simulink model "QuerDynamicModell"  (R2018b)
settings: Solver=VariableStepAuto  StartTime=0.0  StopTime=10.0  RelTol=1e-3
model workspace (MAT data in the model file):
  chStern = 20.5517740291
  controllerActive = 0
  cvStern = 205.517740291
  deltaH = [0 0.02 0.04 0.06 0.08 0.1 0.12 0.14 0.16 0.18 0.2 0.22 0.24 0.26 0.28 0.3 0.32 0.34 0.36 0.38 0.4 0.42 0.44 0.46 0.48 0.5 0.52 0.54 0.56 0.58 0.6 0.62 0.64 0.66 0.68 0.7 0.72 0.74 0.76 0.78 0.8 0.82 0.84 0.86 0.88 0.9 0.92 0.94 0.96 0.98 1 1.02 1.04 1.06 1.08 1.1 1.12 1.14 1.16 1.18 1.2 1.22 1.24 1.26 1.28 1.3 1.32 1.34 1.36 1.38 1.4 1.42 1.44 1.46 1.48 1.5 1.52 1.54 1.56 1.58 1.6 1.62 1.64 1.66 1.68 1.7 1.72 1.74 1.76 1.78 1.8 1.82 1.84 1.86 1.88 1.9 1.92 1.94 1.96 1.98 2 2.02 2.04 2.06 2.08 2.1 2.12 2.14 2.16 2.18 2.2 2.22 2.24 2.26 2.28 2.3 2.32 2.34 2.36 2.38 2.4 2.42 2.44 2.46 2.48 2.5 2.52 2.54 2.56 2.58 2.6 2.62 2.64 2.66 2.68 2.7 2.72 2.74 2.76 2.78 2.8 2.82 2.84 2.86 2.88 2.9 2.92 2.94 2.96 2.98 3 3.02 3.04 3.06 3.08 3.1 3.12 3.14 3.16 3.18 3.2 3.22 3.24 3.26 3.28 3.3 3.32 3.34 3.36 3.38 3.4 3.42 3.44 3.46 3.48 3.5 3.52 3.54 3.56 3.58 3.6 3.62 3.64 3.66 3.68 3.7 3.72 3.74 3.76 3.78 3.8 3.82 3.84 3.86 3.88 3.9 3.92 3.94 3.96 3.98 4 4.02 4.04 4.06 4.08 4.1 4.12 4.14 4.16 4.18 4.2 4.22 4.24 4.26 4.28 4.3 4.32 4.34 4.36 4.38 4.4 4.42 4.44 4.46 4.48 4.5 4.52 4.54 4.56 4.58 4.6 4.62 4.64 4.66 4.68 4.7 4.72 4.74 4.76 4.78 4.8 4.82 4.84 4.86 4.88 4.9 4.92 4.94 4.96 4.98 5 5.02 5.04 5.06 5.08 5.1 5.12 5.14 5.16 5.18 5.2 5.22 5.24 5.26 5.28 5.3 5.32 5.34 5.36 5.38 5.4 5.42 5.44 5.46 5.48 5.5 5.52 5.54 5.56 5.58 5.6 5.62 5.64 5.66 5.68 5.7 5.72 5.74 5.76 5.78 5.8 5.82 5.84 5.86 5.88 5.9 5.92 5.94 5.96 5.98 6]
  g = 9.81
  is = 16
  lh = 1.456
  lv = 1.344
  mDivTheta = 0.574074074074
  r = 1
  v = 100
libraries: simulink x1
settings Model: Creator=User  LastModifiedBy=gregoryseibert
settings DebuggingCC: UnderspecifiedInitializationDetection=Classic

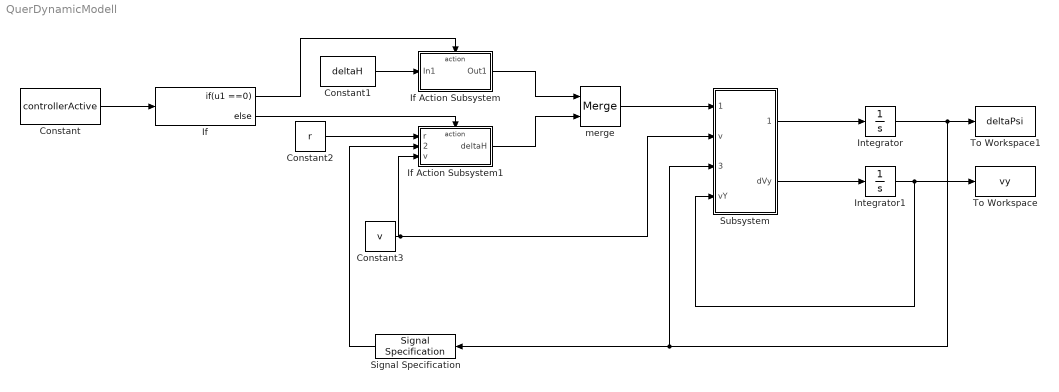
== system QuerDynamicModell ==
  Constant : Constant  Value=controllerActive
  Constant1 : Constant  Value=deltaH
  Constant2 : Constant  Value=r
  Constant3 : Constant  Value=v
  If : If  IfExpression=u1 ==0
  If Action Subsystem : Subsystem  TreatAsAtomicUnit=on
  If Action Subsystem1 : Subsystem  TreatAsAtomicUnit=on
  Integrator : Integrator
  Integrator1 : Integrator
  Signal Specification : SignalSpecification  Dimensions=[301]
  Subsystem : Subsystem
  To Workspace : ToWorkspace  VariableName=vy  SaveFormat=Timeseries  SampleTime=-1
  To Workspace1 : ToWorkspace  VariableName=deltaPsi  SaveFormat=Timeseries  SampleTime=-1
  merge : Merge
  wires:
  Constant/1 -> If/1
  If/1 -> If Action Subsystem/Action
  Constant1/1 -> If Action Subsystem/1(In1)
  If/2 -> If Action Subsystem1/Action
  If Action Subsystem/1(Out1) -> merge/1
  If Action Subsystem1/1(deltaH) -> merge/2
  merge/1 -> Subsystem/1(deltaH)
  Constant2/1 -> If Action Subsystem1/1(r)
  Constant3/1 -> Subsystem/2("v "), If Action Subsystem1/3(v)
  Subsystem/1("delta2Psi ") -> Integrator/1
  Subsystem/2(dVy) -> Integrator1/1
  Integrator/1 -> Subsystem/3(deltaPsi), Signal Specification/1, To Workspace1/1
  Integrator1/1 -> Subsystem/4(vY), To Workspace/1
  Signal Specification/1 -> If Action Subsystem1/2(deltaPsi)

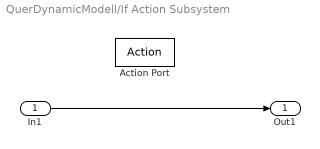
== system QuerDynamicModell/If Action Subsystem ==
  In1 : Inport
  Action Port : ActionPort  ActionType=then
  Out1 : Outport
  wires:
  In1/1 -> Out1/1

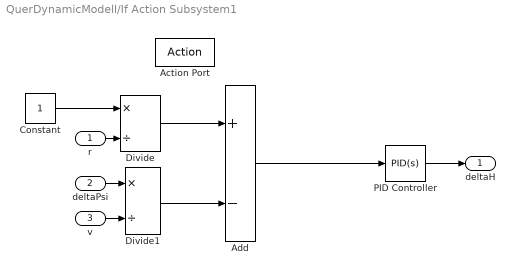
== system QuerDynamicModell/If Action Subsystem1 ==
  r : Inport
  deltaPsi : Inport  Port=2
  v : Inport  Port=3
  Action Port : ActionPort  ActionType=else
  Add : Sum  Inputs=+-
  Constant : Constant
  Divide : Product  Inputs=*/
  Divide1 : Product  Inputs=*/
  PID Controller : simulink/Continuous/PID Controller  Controller=PID  Form=Parallel  TimeDomain=Continuous-time  SampleTime=-1  IntegratorMethod=Forward Euler  FilterMethod=Forward Euler  ControllerParametersSource=internal  P=504.712447211076  I=1502.6695131007  D=0  UseFilter=on  N=100  TunerSelectOption=Transfer Function Based (PID Tuner App)  InitialConditionSource=internal  InitialConditionForIntegrator=0  InitialConditionForFilter=0  DifferentiatorICPrevScaledInput=0  ExternalReset=none  TrackingMode=off  Kt=1  LimitOutput=off  UpperSaturationLimit=inf  LowerSaturationLimit=-inf  LinearizeAsGain=on  AntiWindupMode=none  Kb=1  POutMin=[]  POutMax=[]  IOutMin=[]  IOutMax=[]  DOutMin=[]  DOutMax=[]  NOutMin=[]  NOutMax=[]  SumOutMin=[]  SumOutMax=[]  SaturationOutMin=[]  SaturationOutMax=[]  PParamMin=[]  PParamMax=[]  IParamMin=[]  IParamMax=[]  DParamMin=[]  DParamMax=[]  NParamMin=[]  NParamMax=[]  KbParamMin=[]  KbParamMax=[]  KtParamMin=[]  KtParamMax=[]  KbOutMin=[]  KbOutMax=[]  KtOutMin=[]  KtOutMax=[]  IntegratorOutMin=[]  IntegratorOutMax=[]  FilterOutMin=[]  FilterOutMax=[]  SumI1OutMin=[]  SumI1OutMax=[]  SumI2OutMin=[]  SumI2OutMax=[]  SumI3OutMin=[]  SumI3OutMax=[]  SumI4OutMin=[]  SumI4OutMax=[]  SumDOutMin=[]  SumDOutMax=[]  DifferentiatorOutMin=[]  DifferentiatorOutMax=[]  FilterDiffOutCoefMin=[]  FilterDiffOutCoefMax=[]  ReciprocalOutMin=[]  ReciprocalOutMax=[]  SumDenOutMin=[]  SumDenOutMax=[]  SumNumOutMin=[]  SumNumOutMax=[]  DivideOutMin=[]  DivideOutMax=[]  IntegratorContinuousStateAttributes=''  IntegratorStateMustResolveToSignalObject=off  IntegratorRTWStateStorageClass=Auto  FilterContinuousStateAttributes=''  FilterStateMustResolveToSignalObject=off  FilterRTWStateStorageClass=Auto  ParallelPVariant=InternalParameters  IdealPVariant=Disabled  IVariant=InternalParameters  DVariant=InternalParameters  IntegratorVariant=Continuous  SatVariant=Disabled  AWVariant=Passthrough  PCopyVariant=Disabled  TRVariant=Disabled  FdbkBlocksVariant=Forward  IdealPFdbkVariant=Disabled  SatFdbkVariant=Disabled  DerivativeFilterVariant=ContFilter  NVariant=InternalParameters  NCopyVariant=Disabled  FilterICVariant=InternalICsFilter  IntegratorICVariant=InternalICs  ExternalResetVariant=Disabled  TRSumVariant=Passthrough  SumFdbkVariant=Disabled  SumVariant=Sum_PID
  deltaH : Outport
  wires:
  Constant/1 -> Divide/1
  r/1 -> Divide/2
  deltaPsi/1 -> Divide1/1
  v/1 -> Divide1/2
  Divide/1 -> Add/1
  PID Controller/1 -> deltaH/1
  Add/1 -> PID Controller/1
  Divide1/1 -> Add/2

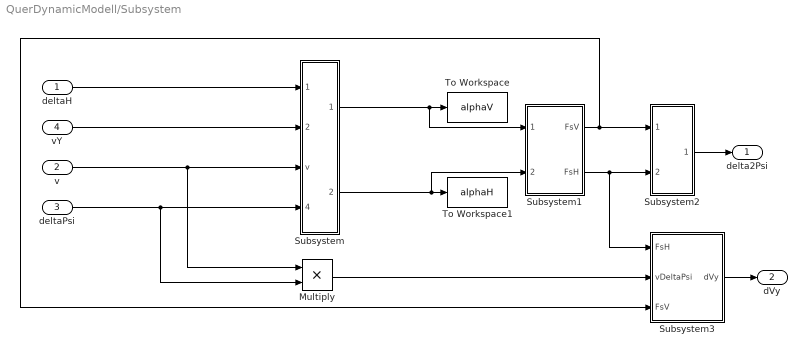
== system QuerDynamicModell/Subsystem ==
  deltaH : Inport
  "v " : Inport  Port=2
  deltaPsi : Inport  Port=3
  vY : Inport  Port=4
  Multiply : Product
  Subsystem : Subsystem
  Subsystem1 : Subsystem
  Subsystem2 : Subsystem
  Subsystem3 : Subsystem
  To Workspace : ToWorkspace  VariableName=alphaV  SaveFormat=Timeseries  SampleTime=-1
  To Workspace1 : ToWorkspace  VariableName=alphaH  SaveFormat=Timeseries  SampleTime=-1
  "delta2Psi " : Outport
  dVy : Outport  Port=2
  wires:
  deltaH/1 -> Subsystem/1(deltaH)
  "v "/1 -> Multiply/1, Subsystem/3(v)
  deltaPsi/1 -> Subsystem/4(deltaPsi), Multiply/2
  Subsystem/1(alphaV) -> Subsystem1/1(alphaV), To Workspace/1
  Subsystem/2(alphaH) -> Subsystem1/2(alphaH), To Workspace1/1
  Subsystem1/1(FsV) -> Subsystem3/3(FsV), Subsystem2/1(FsV)
  Subsystem1/2(FsH) -> Subsystem3/1(FsH), Subsystem2/2(FsH)
  Subsystem2/1(delta2Psi) -> "delta2Psi "/1
  Subsystem3/1("dVy ") -> dVy/1
  Multiply/1 -> Subsystem3/2(vDeltaPsi)
  vY/1 -> Subsystem/2(vY)

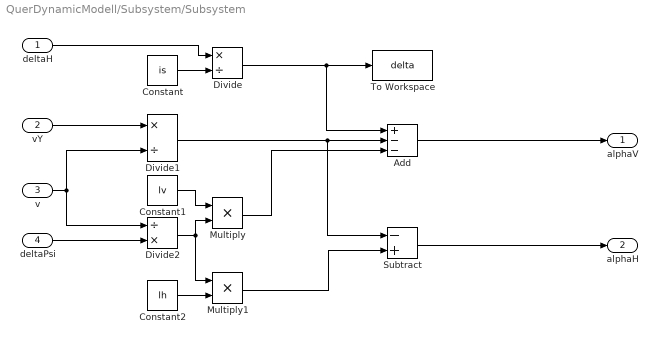
== system QuerDynamicModell/Subsystem/Subsystem ==
  deltaH : Inport
  vY : Inport  Port=2
  v : Inport  Port=3
  deltaPsi : Inport  Port=4
  Add : Sum  Inputs=+--
  Constant : Constant  Value=is
  Constant1 : Constant  Value=lv
  Constant2 : Constant  Value=lh
  Divide : Product  Inputs=*/
  Divide1 : Product  Inputs=*/
  Divide2 : Product  Inputs=/*
  Multiply : Product
  Multiply1 : Product
  Subtract : Sum  Inputs=-+
  To Workspace : ToWorkspace  VariableName=delta  SaveFormat=Timeseries  SampleTime=-1
  alphaV : Outport
  alphaH : Outport  Port=2
  wires:
  Subtract/1 -> alphaH/1
  v/1 -> Divide1/2, Divide2/1
  Add/1 -> alphaV/1
  Constant/1 -> Divide/2
  Divide2/1 -> Multiply1/1, Multiply/2
  vY/1 -> Divide1/1
  deltaPsi/1 -> Divide2/2
  Constant1/1 -> Multiply/1
  Constant2/1 -> Multiply1/2
  Multiply1/1 -> Subtract/2
  deltaH/1 -> Divide/1
  Divide/1 -> Add/1, To Workspace/1
  Divide1/1 -> Add/2, Subtract/1
  Multiply/1 -> Add/3

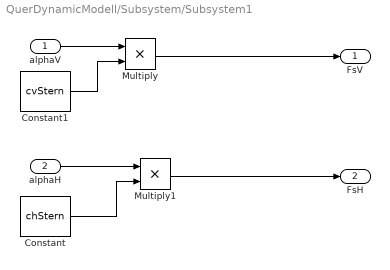
== system QuerDynamicModell/Subsystem/Subsystem1 ==
  alphaV : Inport
  alphaH : Inport  Port=2
  Constant : Constant  Value=chStern
  Constant1 : Constant  Value=cvStern
  Multiply : Product
  Multiply1 : Product
  FsV : Outport
  FsH : Outport  Port=2
  wires:
  alphaH/1 -> Multiply1/1
  Constant/1 -> Multiply1/2
  alphaV/1 -> Multiply/1
  Constant1/1 -> Multiply/2
  Multiply/1 -> FsV/1
  Multiply1/1 -> FsH/1

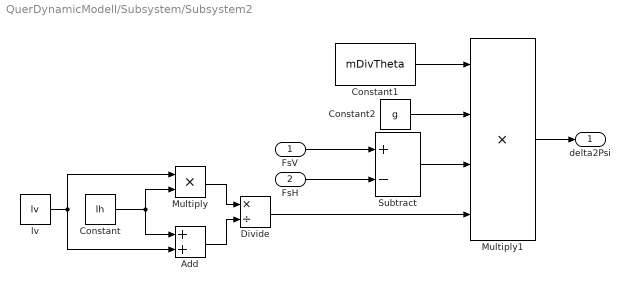
== system QuerDynamicModell/Subsystem/Subsystem2 ==
  FsV : Inport
  FsH : Inport  Port=2
  Add : Sum
  Constant : Constant  Value=lh
  Constant1 : Constant  Value=mDivTheta
  Constant2 : Constant  Value=g
  Divide : Product  Inputs=*/
  Multiply : Product
  Multiply1 : Product  Inputs=4
  Subtract : Sum  Inputs=+-
  lv : Constant  Value=lv
  delta2Psi : Outport
  wires:
  FsV/1 -> Subtract/1
  Constant/1 -> Add/1, Multiply/2
  lv/1 -> Add/2, Multiply/1
  Multiply/1 -> Divide/1
  Add/1 -> Divide/2
  Constant1/1 -> Multiply1/1
  Constant2/1 -> Multiply1/2
  FsH/1 -> Subtract/2
  Subtract/1 -> Multiply1/3
  Divide/1 -> Multiply1/4
  Multiply1/1 -> delta2Psi/1

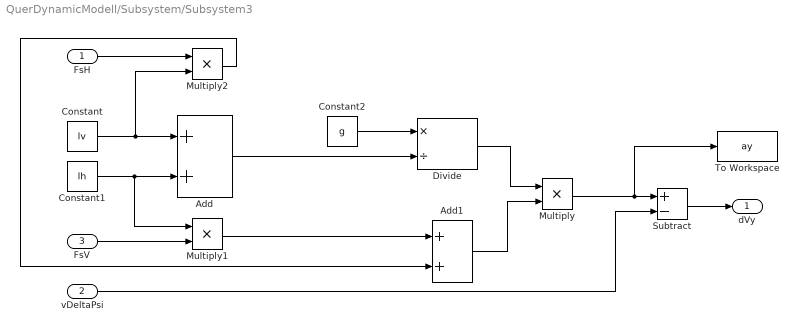
== system QuerDynamicModell/Subsystem/Subsystem3 ==
  FsH : Inport
  vDeltaPsi : Inport  Port=2
  FsV : Inport  Port=3
  Add : Sum
  Add1 : Sum
  Constant : Constant  Value=lv
  Constant1 : Constant  Value=lh
  Constant2 : Constant  Value=g
  Divide : Product  Inputs=*/
  Multiply : Product
  Multiply1 : Product
  Multiply2 : Product
  Subtract : Sum  Inputs=+-
  To Workspace : ToWorkspace  VariableName=ay  SaveFormat=Timeseries  SampleTime=-1
  "dVy " : Outport
  wires:
  Constant1/1 -> Multiply1/1, Add/2
  Constant/1 -> Multiply2/2, Add/1
  Add/1 -> Divide/2
  Constant2/1 -> Divide/1
  FsV/1 -> Multiply1/2
  FsH/1 -> Multiply2/1
  Multiply2/1 -> Add1/2
  Multiply1/1 -> Add1/1
  Divide/1 -> Multiply/1
  Add1/1 -> Multiply/2
  Multiply/1 -> To Workspace/1, Subtract/1
  vDeltaPsi/1 -> Subtract/2
  Subtract/1 -> "dVy "/1
